simulink model "A310_hj"  (R2021b)
settings: Solver=FixedStepDiscrete  StartTime=0.0  StopTime=TSim  RelTol=1e-3
model workspace (MAT data in the model file):
  LengthOfPilot = 16000
undefined symbols (not defined in the file or in its folder): freqz, fs, lenPilotSig
libraries: dspswit3 x2, dspsrcs4 x2, dspspect3 x1, matrix_library x1, dspadpt3 x1, dspsnks4 x1
settings Model: Creator=Feldes  LastModifiedBy=Feldes
settings SolverCC: AlgebraicLoopSolver=TrustRegion  AutoInsertRateTranBlk=on
settings DataIOCC: LimitDataPoints=on  SaveOutput=off  SignalLogging=off  SaveTime=off
settings OptimizationCC: LifeSpan=inf  SimCompilerOptimization=on
settings DebuggingCC: AlgebraicLoopMsg=error  SingleTaskRateTransMsg=error  AllowSymbolicDim=off  SFUnexpectedBacktrackingDiag=warning  SFNoUnconditionalDefaultTransitionDiag=warning  SFExecutionAtInitializationDiag=none  SFMachineParentedDataDiag=warning  ArithmeticOperatorsInVariantConditions=warning
settings SFSimCC: SimUseLocalCustomCode=off  CustomCodeUndefinedFunction=UseInterfaceOnly
settings RTWCC: RTWUseLocalCustomCode=off
settings CodeAppCC: StateflowObjectComments=on
settings GRTTargetCC: TargetLangStandard=C89/C90 (ANSI)
settings ConfigComp: CovMetricSettings=dw  CovSaveCumulativeToWorkspaceVar=on  CovSaveSingleToWorkspaceVar=on  CovExternalEMLEnable=off  CovSFcnEnable=off

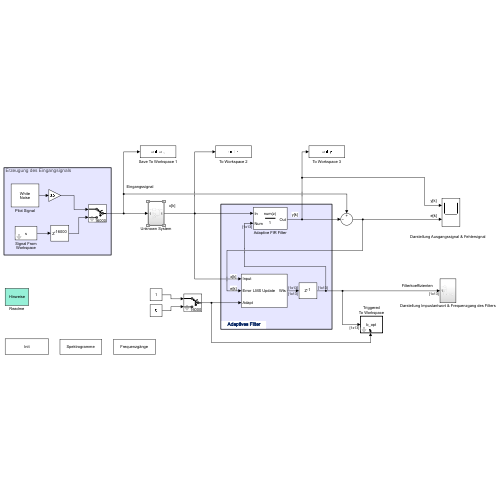
[thumbnail: Simulink's stored preview of the top-level diagram]
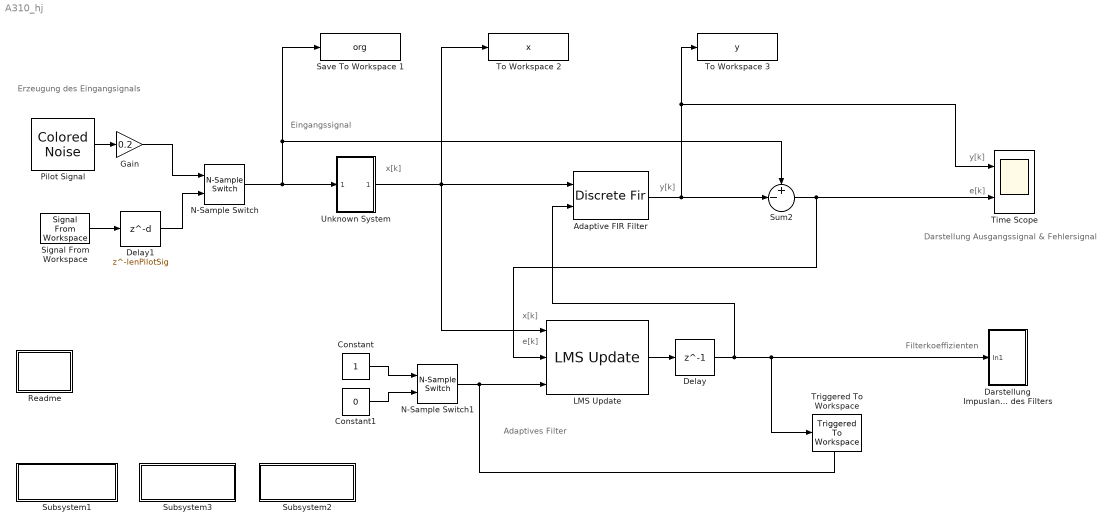
== system A310_hj ==
  note: Erzeugung des Eingangsignals
  note: Adaptives Filter
  note: e[k]
  note: y[k]
  note: Darstellung Ausgangssignal & Fehlersignal
  note: Filterkoeffizienten
  note: x[k]
  note: e[k]
  note: y[k]
  note: x[k]
  note: Eingangssignal
  Adaptive FIR Filter : DiscreteFir  CoefSource=Input port  InputProcessing=Columns as channels (frame based)
      settings: InputPortMap=u0,u1
  Constant : Constant
  Constant1 : Constant  Value=0
  Darstellung Impuslantwort & Frequenzgang des Filters : Subsystem
  Delay : Delay  DelayLength=1  InputProcessing=Columns as channels (frame based)
  Delay1 : Delay  DelayLength=lenPilotSig  InputProcessing=Columns as channels (frame based)
  Gain : Gain  Gain=0.2
  LMS Update : dspadpt3/LMS Update  Method=LMS  Length=13  StepSizeSource=Property  StepSize=0.00333  LeakageFactor=1.0  InitialConditions=0  EnableAdaptInput=on  EnableResetInput=off  SimulateUsing=Code generation
      settings: SourceProductBaseCode=DS
  N-Sample Switch : dspswit3/N-Sample Switch  N=lenPilotSig  reset=off  TriggerType=Rising edge  Ts=1/fs
      settings: SourceProductBaseCode=DS
  N-Sample Switch1 : dspswit3/N-Sample Switch  N=lenPilotSig  reset=off  TriggerType=Rising edge  Ts=1/fs
      settings: SourceProductBaseCode=DS
  Pilot Signal : dspsrcs4/Colored Noise  Color=white  InverseFrequencyPower=1  BoundedOutput=on  NumChannels=1  OutputDataType=double  SamplesPerFrame=1  SampleTime=1/fs  RandomStream=mt19937ar with seed  Seed=67  SimulateUsing=Interpreted execution
      settings: SourceProductBaseCode=DS
  Readme : Subsystem
      mask Display: disp('Hinweise')
  Save To Workspace 1 : ToWorkspace  VariableName=org  SampleTime=-1
      settings: Save2DSignal=2-D array (concatenate along first dimension)
  Signal From Workspace : dspsrcs4/Signal From Workspace  X=s  Ts=1/fs  nsamps=1  OutputAfterFinalValue=Setting to zero  ignoreOrWarnInputAndFrameLengths=off  OutputFrames=off
  Subsystem1 : Subsystem
      settings: OpenFcn=|
      | lenPilotSig= 16000;
      | [s,fs]=audioread('bbauer8s.wav');
      | TSim =lenPilotSig/fs + length(s)/fs;
      | pauseTimes=[0.05 0.1 0.2 0.4 0.8 1.4 2];
      mask Display: disp('Init')
  Subsystem2 : Subsystem
      settings: OpenFcn=|
      | if exist('out','var'), freqResponse_Hall();
      | else errordlg('You must run the simulation first.','DSP Blockset Demo Error'); end
      mask Display: disp('Frequenzgänge')
  Subsystem3 : Subsystem
      settings: OpenFcn=|
      | if exist('out','var'), SpectrogramExample(out.org, fs); SpectrogramExample(out.x, fs); SpectrogramExample(out.y, fs);
      | else errordlg('You must run the simulation first.','DSP Blockset Demo Error'); end
      mask Display: disp('Spektrogramme')
  Sum2 : Sum  Inputs=+-|  InputSameDT=on  SaturateOnIntegerOverflow=on  OutDataTypeStr=Inherit: Same as first input
  Time Scope : Scope  NumInputPorts=2
  To Workspace 2 : ToWorkspace  VariableName=x  SampleTime=-1
      settings: Save2DSignal=2-D array (concatenate along first dimension)
  To Workspace 3 : ToWorkspace  VariableName=y  SampleTime=-1
      settings: Save2DSignal=2-D array (concatenate along first dimension)
  Triggered To Workspace : dspsnks4/Triggered To Workspace  TriggerType=Falling edge  VariableName=b_opt  Buffer=1000  Save2DMode=2-D array (concatenate along first dimension)
      settings: SourceProductBaseCode=DS  FixptAsFi=off
  Unknown System : Subsystem
  wires:
  Sum2/1 -> LMS Update/2, Time Scope/2
  LMS Update/1 -> Delay/1
  N-Sample Switch1/1 -> Triggered To Workspace/Trigger, LMS Update/3
  Constant/1 -> N-Sample Switch1/1
  Constant1/1 -> N-Sample Switch1/2
  Delay/1 -> Triggered To Workspace/1, Darstellung Impuslantwort & Frequenzgang des Filters/1(In1), Adaptive FIR Filter/2
  Adaptive FIR Filter/1 -> Time Scope/1, To Workspace 3/1, Sum2/2
  Unknown System/1(Out1) -> Adaptive FIR Filter/1, LMS Update/1, To Workspace 2/1
  N-Sample Switch/1 -> Save To Workspace 1/1, Sum2/1, Unknown System/1(In1)
  Pilot Signal/1 -> Gain/1
  Gain/1 -> N-Sample Switch/1
  Signal From Workspace/1 -> Delay1/1
  Delay1/1 -> N-Sample Switch/2

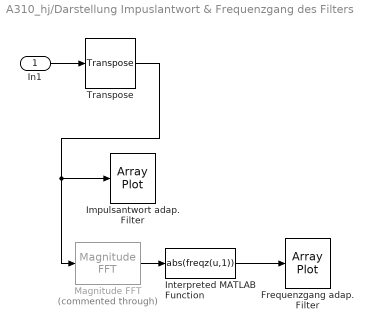
== system A310_hj/Darstellung Impuslantwort & Frequenzgang des Filters ==
  In1 : Inport
  Frequenzgang adap. Filter : ArrayPlot  WindowPosition=[1057.000000,499.000000,611.000000,454.000000,]  Visible=on  SampleIncrement=7.8125  YScale=Log  PlotType=Line  AxesScaling=Manual  XLabel=Frequency (Hz)  YLimits=[0.001,10]
  Impulsantwort adap. Filter : ArrayPlot  WindowPosition=[1045.000000,42.000000,619.000000,474.000000,]  Visible=on  AxesScaling=Manual  YLimits=[-1,1.2]
  Interpreted MATLAB Function : MATLABFcn  MATLABFcn=abs(freqz(u,1))
  Magnitude FFT : dspspect3/Magnitude FFT  Commented=through  mag_or_magsq=Magnitude  FFTImplementation=Auto  fftLenInherit=off  fftsize=256  WrapInput=on
      settings: SourceProductBaseCode=DS
  Transpose : matrix_library/Transpose
      settings: SourceProductBaseCode=SL
  wires:
  Transpose/1 -> Magnitude FFT/1, Impulsantwort adap. Filter/1
  Interpreted MATLAB Function/1 -> Frequenzgang adap. Filter/1
  In1/1 -> Transpose/1
  Magnitude FFT/1 -> Interpreted MATLAB Function/1

== system A310_hj/Readme ==
  note: h) Aktivieren der additiven Störung durch Doppelklick auf unbekanntes System und ändern des Faktors auf 1
      |
      | i) Ändern der Koeffizientenanzahl durch Doppelklick auf LMS-Update-Block und editieren von Filterlength
      |
      | Ändern der Länge des Pilotsignals durch ändern der Variablen lenPilotSig im Workspace

== system A310_hj/Subsystem1 ==

== system A310_hj/Subsystem2 ==

== system A310_hj/Subsystem3 ==

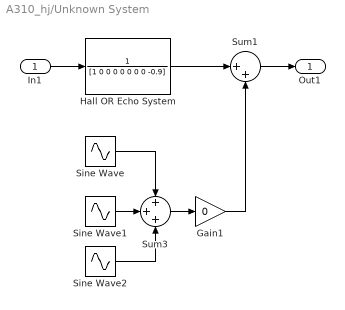
== system A310_hj/Unknown System ==
  In1 : Inport
  Gain1 : Gain  Gain=0
  Hall OR Echo System : DiscreteFilter  Numerator=1  Denominator=[1 0 0 0 0 0 0 0 -0.9]  InputProcessing=Columns as channels (frame based)  FilterStructure=Direct form II transposed  a0EqualsOne=on
  Sine Wave : Sin  Amplitude=1./7.  Frequency=24.9/40*pi*8000  SampleTime=1/fs
  Sine Wave1 : Sin  Amplitude=1./7.  Frequency=25/40*pi*8000  SampleTime=1/fs
  Sine Wave2 : Sin  Amplitude=1./7.  Frequency=25.1/40*pi*8000  SampleTime=1/fs
  Sum1 : Sum  Inputs=|++  InputSameDT=on  SaturateOnIntegerOverflow=on  OutDataTypeStr=Inherit: Same as first input
  Sum3 : Sum  Inputs=+++  InputSameDT=on  SaturateOnIntegerOverflow=on  OutDataTypeStr=Inherit: Same as first input
  Out1 : Outport
  wires:
  Sum1/1 -> Out1/1
  Hall OR Echo System/1 -> Sum1/1
  Gain1/1 -> Sum1/2
  Sine Wave/1 -> Sum3/1
  Sum3/1 -> Gain1/1
  Sine Wave1/1 -> Sum3/2
  Sine Wave2/1 -> Sum3/3
  In1/1 -> Hall OR Echo System/1
